simulink model "Lidar_System_July03_v2_noSave"  (Simulink 7.3)
settings: Solver=FixedStepDiscrete  StartTime=0.0  StopTime=inf  FixedStep=0.1  MaxStep=0.2  RelTol=1e-3
undefined symbols (not defined in the file): strel
libraries: dspmtrx3 x86, simulink x64, dspstat3 x37, vipstatistics x15, vipmorphops x15
(part 1 of 8)
settings Model: Creator=gclayton  LastModifiedBy=wildcat
settings DebuggingCC: InheritedTsInSrcMsg=none
settings RTWCC: SystemTargetFile=rlnx.tlc  GenCodeOnly=on  TemplateMakefile=rlnx_ubuntu.tmf  Description=Linux Real-Time Target  ProcessScript=rlnx_make_rtw_hook
settings RTWCC: CustomInclude=|
  | /usr/local/include/opencv/
  | /usr/local/include/
settings CodeAppCC: GenerateComments=off  SimulinkBlockComments=off
settings STFCustomTargetCC: ModelReferenceCompliant=off  MatFileLogging=on  SystemTargetFile=rlnx.tlc
settings GRTTargetCC: ModelReferenceCompliant=off  ParMdlRefBuildCompliant=off  CompOptLevelCompliant=off
settings CustomProperty: DataType=string  Value="-lm -ldl /usr/local/lib/libopencv_highgui.so.2.4 /usr/local/lib/libopencv_core.so.2.4 /usr/local/lib/libopencv_imgproc.so.2.4  -lc_urg -lc_urg_connection -lc_urg_system -lphidget21 -llcm"
settings EnumStrPairs: String=PC

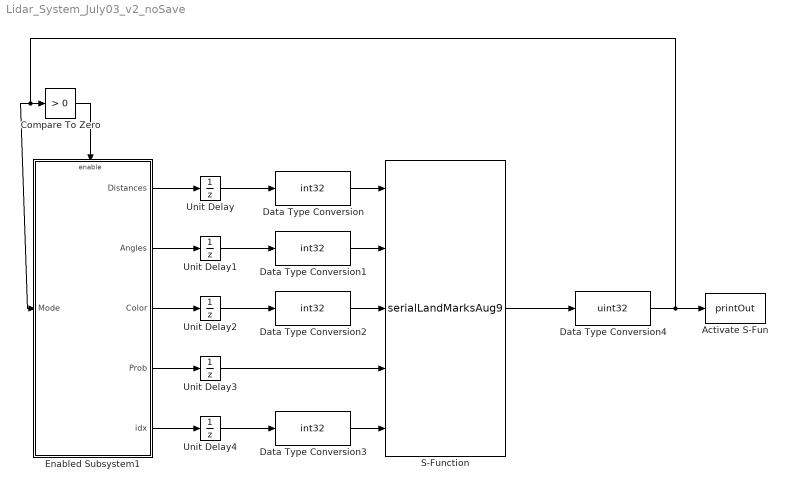
== system Lidar_System_July03_v2_noSave ==
  Activate S-Fun : S-Function  FunctionName=printOut  EnableBusSupport=off
  Compare To Zero : simulink/Logic and Bit Operations/Compare To Zero  SystemSampleTime=-1  relop=>  LogicOutDataTypeMode=uint8  ZeroCross=off
  Data Type Conversion{,1..3} (4 alike) : DataTypeConversion  OutDataTypeMode=int32  OutDataType=fixdt(1, 16)  OutScaling=2^0  OutDataTypeStr=int32
  Data Type Conversion4 : DataTypeConversion  OutDataTypeMode=uint32  OutDataType=fixdt(1, 16)  OutScaling=2^0  OutDataTypeStr=uint32
  Enabled Subsystem1 : Subsystem  TreatAsAtomicUnit=on
  S-Function : S-Function  FunctionName=serialLandMarksAug9  EnableBusSupport=off
  Unit Delay : UnitDelay  X0=zeros(1,12)  SampleTime=-1
  Unit Delay1 : UnitDelay  X0=zeros(1,12)  SampleTime=-1
  Unit Delay2 : UnitDelay  X0=zeros(4,1)  SampleTime=-1
  Unit Delay3 : UnitDelay  X0=zeros(4,1)  SampleTime=-1
  Unit Delay4 : UnitDelay  X0=zeros(4,1)  SampleTime=-1
  wires:
  Compare To Zero/1 -> Enabled Subsystem1/Enable
  Data Type Conversion4/1 -> Activate S-Fun/1, Compare To Zero/1, Enabled Subsystem1/1(Mode)
  S-Function/1 -> Data Type Conversion4/1
  Enabled Subsystem1/2(Angles) -> Unit Delay1/1
  Enabled Subsystem1/1(Distances) -> Unit Delay/1
  Enabled Subsystem1/3(Color) -> Unit Delay2/1
  Enabled Subsystem1/4(Prob) -> Unit Delay3/1
  Enabled Subsystem1/5(idx) -> Unit Delay4/1
  Unit Delay/1 -> Data Type Conversion/1
  Unit Delay1/1 -> Data Type Conversion1/1
  Unit Delay2/1 -> Data Type Conversion2/1
  Unit Delay4/1 -> Data Type Conversion3/1
  Data Type Conversion/1 -> S-Function/1
  Data Type Conversion1/1 -> S-Function/2
  Data Type Conversion2/1 -> S-Function/3
  Unit Delay3/1 -> S-Function/4
  Data Type Conversion3/1 -> S-Function/5

== system Lidar_System_July03_v2_noSave/Enabled Subsystem1 ==
  Mode : Inport  OutDataType=fixdt(1, 16)  OutScaling=2^0
  Enable : EnablePort
  Data Type Conversion : DataTypeConversion  OutDataTypeMode=int32  OutDataType=fixdt(1, 16)  OutScaling=2^0  OutDataTypeStr=int32
  Down Angle : Constant  Value=-25  OutDataType=fixdt(1, 16)  OutScaling=2^0
  Embedded MATLAB Function : Stateflow chart  TreatAsAtomicUnit=on
  Perception : Subsystem  TreatAsAtomicUnit=on
  S-Function : S-Function  FunctionName=TT_pot_readerV4  EnableBusSupport=off
  Scan Number (max 65) : Constant  Value=65  OutDataType=fixdt(1, 16)  OutScaling=2^0
  Sensing : S-Function  FunctionName=lidarCam_Select_June30_15  EnableBusSupport=off
  Sensor Enable : Stateflow chart  TreatAsAtomicUnit=on
  Stepper Speed and Postion  Calculation : Stateflow chart  TreatAsAtomicUnit=on
  Up Angle : Constant  Value=30  OutDataType=fixdt(1, 16)  OutScaling=2^0
  Distances : Outport  OutDataType=fixdt(1, 16)  OutScaling=2^0
  Angles : Outport  Port=2  OutDataType=fixdt(1, 16)  OutScaling=2^0
  Color : Outport  Port=3  OutDataType=fixdt(1, 16)  OutScaling=2^0
  Prob : Outport  Port=4  OutDataType=fixdt(1, 16)  OutScaling=2^0
  idx : Outport  Port=5  OutDataType=fixdt(1, 16)  OutScaling=2^0
  wires:
  Embedded MATLAB Function/1(yn) -> Perception/Enable
  Sensing/1 -> Perception/2(LidarData)
  Sensing/5 -> Perception/6(UpDown)
  Sensing/2 -> Perception/3(Red)
  Sensing/3 -> Perception/4(Green)
  Sensing/4 -> Perception/5(Blue)
  Mode/1 -> Perception/1(Mode), Sensor Enable/1(mode)
  Down Angle/1 -> Stepper Speed and Postion  Calculation/2(DownAngle)
  Up Angle/1 -> Stepper Speed and Postion  Calculation/1(UpAngle)
  Scan Number (max 65)/1 -> Stepper Speed and Postion  Calculation/3(Scans)
  Stepper Speed and Postion  Calculation/1(Speed) -> Sensing/3
  Stepper Speed and Postion  Calculation/2(Upos) -> Sensing/4
  Stepper Speed and Postion  Calculation/3(Dpos) -> Sensing/5
  Stepper Speed and Postion  Calculation/4(ScanNum) -> Sensing/6
  S-Function/1 -> Embedded MATLAB Function/1(potVal), Sensing/2
  Sensor Enable/1(choice) -> Data Type Conversion/1
  Data Type Conversion/1 -> Sensing/1
  Perception/1(Distances) -> Distances/1
  Perception/2(Angles) -> Angles/1
  Perception/3(Color) -> Color/1
  Perception/4(Prob) -> Prob/1
  Perception/5(idx) -> idx/1

== system Lidar_System_July03_v2_noSave/Enabled Subsystem1/Perception ==
  Mode : Inport  OutDataType=fixdt(1, 16)  OutScaling=2^0
  LidarData : Inport  Port=2  OutDataType=fixdt(1, 16)  OutScaling=2^0
  Red : Inport  Port=3  OutDataType=fixdt(1, 16)  OutScaling=2^0
  Green : Inport  Port=4  OutDataType=fixdt(1, 16)  OutScaling=2^0
  Blue : Inport  Port=5  OutDataType=fixdt(1, 16)  OutScaling=2^0
  UpDown : Inport  Port=6  OutDataType=fixdt(1, 16)  OutScaling=2^0
  Enable : EnablePort
  Bus Creator : BusCreator  Inputs=3
  Color Analysis : Subsystem
  Detect Landmarks : Subsystem
  Lidar data selector : Stateflow chart  TreatAsAtomicUnit=on
  Match Landmarks : Stateflow chart  TreatAsAtomicUnit=on
  Raster Image : Stateflow chart  TreatAsAtomicUnit=on
  Raster to UV scatter : Stateflow chart  TreatAsAtomicUnit=on
  Raster to UV scatter1 : Stateflow chart  TreatAsAtomicUnit=on
  S-Function4 : S-Function  FunctionName=rgbtohsv_sfunV2  EnableBusSupport=off
  Distances : Outport  OutDataType=fixdt(1, 16)  OutScaling=2^0
  Angles : Outport  Port=2  OutDataType=fixdt(1, 16)  OutScaling=2^0
  Color : Outport  Port=3  OutDataType=fixdt(1, 16)  OutScaling=2^0
  Prob : Outport  Port=4  OutDataType=fixdt(1, 16)  OutScaling=2^0
  idx : Outport  Port=5  OutDataType=fixdt(1, 16)  OutScaling=2^0
  wires:
  Lidar data selector/1(lidarOut) -> Raster Image/1(lidarData)
  Red/1 -> S-Function4/1
  Green/1 -> S-Function4/2
  Blue/1 -> S-Function4/3
  LidarData/1 -> Lidar data selector/1(lidarIn)
  S-Function4/1 -> Bus Creator/1  "H"
  S-Function4/2 -> Bus Creator/2  "S"
  S-Function4/3 -> Bus Creator/3  "V"
  Bus Creator/1 -> Color Analysis/3(HSV)
  Raster to UV scatter/1(depthImage) -> Color Analysis/2(uv_d)
  Mode/1 -> Color Analysis/1(Mode)
  Color Analysis/2(Prob) -> Prob/1
  Color Analysis/1(Color) -> Color/1
  Color Analysis/3(im_distances) -> Match Landmarks/1(im_distances)
  Color Analysis/4(im_angles) -> Match Landmarks/2(im_angles)
  Detect Landmarks/1(Distances) -> Match Landmarks/3(Distances)
  Detect Landmarks/2(Angles) -> Match Landmarks/4(Angles)
  Raster Image/1(dist_image) -> Raster to UV scatter1/1(DistIM), Detect Landmarks/1(dist_im)
  Raster to UV scatter1/1(scanAngle) -> Raster to UV scatter/1(scanAngle)
  Raster to UV scatter1/2(gimbalAngle) -> Raster to UV scatter/2(gimbalAngle)
  Raster to UV scatter1/3(range) -> Raster to UV scatter/3(range)
  Match Landmarks/1(idx) -> idx/1
  Match Landmarks/2(distances) -> Distances/1
  Match Landmarks/3(angles) -> Angles/1
  UpDown/1 -> Raster to UV scatter/4(upScan), Raster Image/2(UpDown)

== system Lidar_System_July03_v2_noSave/Enabled Subsystem1/Perception/Color Analysis ==
  Mode : Inport  OutDataType=fixdt(1, 16)  OutScaling=2^0
  uv_d : Inport  Port=2  OutDataType=fixdt(1, 16)  OutScaling=2^0
  HSV : Inport  Port=3  OutDataType=fixdt(1, 16)  OutScaling=2^0
  Acoustics (Empty) : Subsystem  TreatAsAtomicUnit=on
  Bus Selector : BusSelector  OutputSignals=Color,Prob,im_distances,im_angles
  Find Can Buoys : Subsystem  TreatAsAtomicUnit=on
  Light Buoy : Subsystem  TreatAsAtomicUnit=on
  Multiport Switch : MultiPortSwitch  Inputs=5  OutDataType=fixdt(1, 16)  OutScaling=2^0
  No Color Analysis1 : Subsystem  TreatAsAtomicUnit=on
  Switch Case : SwitchCase  CaseConditions={1,2,3,4}
  Template Matching (Docking) : Subsystem  TreatAsAtomicUnit=on
  Color : Outport  OutDataType=fixdt(1, 16)  OutScaling=2^0
  Prob : Outport  Port=2  OutDataType=fixdt(1, 16)  OutScaling=2^0
  im_distances : Outport  Port=3  OutDataType=fixdt(1, 16)  OutScaling=2^0
  im_angles : Outport  Port=4  OutDataType=fixdt(1, 16)  OutScaling=2^0
  wires:
  Mode/1 -> Switch Case/1, Multiport Switch/1, Template Matching (Docking)/3(mode)
  Find Can Buoys/1(Output) -> Multiport Switch/2
  Acoustics (Empty)/1(Output) -> Multiport Switch/3
  Bus Selector/1 -> Color/1  "<Color>"
  Bus Selector/2 -> Prob/1  "<Prob>"
  Bus Selector/3 -> im_distances/1  "<im_distances>"
  Bus Selector/4 -> im_angles/1  "<im_angles>"
  Template Matching (Docking)/1(Output) -> Multiport Switch/6
  Multiport Switch/1 -> Bus Selector/1
  Light Buoy/1(Output) -> Multiport Switch/4
  No Color Analysis1/1(Output) -> Multiport Switch/5
  Switch Case/1 -> Find Can Buoys/Action
  Switch Case/2 -> Acoustics (Empty)/Action
  Switch Case/3 -> Light Buoy/Action
  Switch Case/4 -> No Color Analysis1/Action
  uv_d/1 -> Find Can Buoys/1(uv_d), Acoustics (Empty)/1(uv_d), Light Buoy/1(uv_d), No Color Analysis1/1(uv_d), Template Matching (Docking)/1(uv_d)
  HSV/1 -> Light Buoy/2(HSV), No Color Analysis1/2(HSV), Template Matching (Docking)/2(HSV), Acoustics (Empty)/2(HSV), Find Can Buoys/2(HSV)
  Switch Case/5 -> Template Matching (Docking)/Action

== system Lidar_System_July03_v2_noSave/Enabled Subsystem1/Perception/Detect Landmarks ==
  dist_im : Inport  OutDataType=fixdt(1, 16)  OutScaling=2^0
  Blob Analysis : vipstatistics/Blob Analysis  Tag=vipblks_row_conv  DialogController=vipDDGCreate  DialogControllerArgs=DataTag51  area=off  centroid=on  bBox=on  majorAxis=off  minorAxis=off  angle=off  eccentricity=off  equivDiameterSq=off  extent=off  perimeter=off  maxBlobs=12  warnIfNumBlobsExceeded=on  isCount=off  useMinArea=on  minArea=30  useMaxArea=off  maxArea=intmax('uint32')  excludeBorderBlob=on  outDT=double  isOutVarDim=off  isFill=on  fillValues=-1  conn=8  isLabel=off  outputMode=Binary point scaling  outputWordLength=32  outputFracLength=16  firstCoeffMode=Binary point scaling  firstCoeffWordLength=16  firstCoeffFracLength=14  secondCoeffMode=Binary point scaling  secondCoeffWordLength=32  secondCoeffFracLength=16  accumMode=Binary point scaling  accumWordLength=32  accumFracLength=0  prodOutputMode=Binary point scaling  prodOutputWordLength=32  prodOutputFracLength=16  roundingMode=Floor  overflowMode=off
  Closing : vipmorphops/Closing  nhoodsrc=Specify via dialog  strel=strel('rectangle',[5 7])
  Embedded MATLAB Function1 : Stateflow chart  TreatAsAtomicUnit=on
  Logical Operator : Logic  AllPortsSameDT=off  OutDataTypeMode=boolean  LogicDataType=fixdt(0, 8)  OutDataTypeStr=boolean
  Max Thresh : simulink/Logic and Bit Operations/Compare To Constant  SystemSampleTime=-1  relop=<=  const=10000  LogicOutDataTypeMode=boolean  ZeroCross=off
  Min Thresh (removes pontoons) : simulink/Logic and Bit Operations/Compare To Constant  SystemSampleTime=-1  relop=>  const=2000  LogicOutDataTypeMode=boolean  ZeroCross=off
  Distances : Outport  OutDataType=fixdt(1, 16)  OutScaling=2^0
  Angles : Outport  Port=2  OutDataType=fixdt(1, 16)  OutScaling=2^0
  wires:
  Max Thresh/1 -> Logical Operator/1
  Min Thresh (removes pontoons)/1 -> Logical Operator/2
  dist_im/1 -> Max Thresh/1, Min Thresh (removes pontoons)/1, Embedded MATLAB Function1/4(dist_im)
  Embedded MATLAB Function1/1(Distances) -> Distances/1
  Embedded MATLAB Function1/2(Angles) -> Angles/1
  Logical Operator/1 -> Closing/1, Embedded MATLAB Function1/3(BW)
  Closing/1 -> Blob Analysis/1
  Blob Analysis/1 -> Embedded MATLAB Function1/1(centroid)
  Blob Analysis/2 -> Embedded MATLAB Function1/2(bbox)

== system Lidar_System_July03_v2_noSave/Enabled Subsystem1/Perception/Color Analysis/Acoustics (Empty) ==
  uv_d : Inport  OutDataType=fixdt(1, 16)  OutScaling=2^0
  HSV : Inport  Port=2  OutDataType=fixdt(1, 16)  OutScaling=2^0
  Action Port : ActionPort  ActionType=case
  Bus Creator : BusCreator
  Constant{,1..3} (4 alike) : Constant  Value=zeros(4,1)  OutDataType=fixdt(1, 16)  OutScaling=2^0
  Terminator : Terminator
  Terminator1 : Terminator
  Output : Outport  OutDataType=fixdt(1, 16)  OutScaling=2^0
  wires:
  uv_d/1 -> Terminator/1
  HSV/1 -> Terminator1/1
  Bus Creator/1 -> Output/1
  Constant3/1 -> Bus Creator/4  "im_angles"
  Constant2/1 -> Bus Creator/3  "im_distances"
  Constant1/1 -> Bus Creator/2  "Prob"
  Constant/1 -> Bus Creator/1  "Color"

== system Lidar_System_July03_v2_noSave/Enabled Subsystem1/Perception/Color Analysis/Find Can Buoys ==
  uv_d : Inport  OutDataType=fixdt(1, 16)  OutScaling=2^0
  HSV : Inport  Port=2  OutDataType=fixdt(1, 16)  OutScaling=2^0
  Action Port : ActionPort  ActionType=case
  Blob Analysis : vipstatistics/Blob Analysis  Tag=vipblks_row_conv  DialogController=vipDDGCreate  DialogControllerArgs=DataTag0  area=off  centroid=on  bBox=on  majorAxis=off  minorAxis=off  angle=off  eccentricity=off  equivDiameterSq=off  extent=off  perimeter=off  maxBlobs=12  warnIfNumBlobsExceeded=on  isCount=off  useMinArea=on  minArea=20  useMaxArea=off  maxArea=intmax('uint32')  excludeBorderBlob=on  outDT=double  isOutVarDim=off  isFill=on  fillValues=-1  conn=8  isLabel=off  outputMode=Binary point scaling  outputWordLength=32  outputFracLength=16  firstCoeffMode=Binary point scaling  firstCoeffWordLength=16  firstCoeffFracLength=14  secondCoeffMode=Binary point scaling  secondCoeffWordLength=32  secondCoeffFracLength=16  accumMode=Binary point scaling  accumWordLength=32  accumFracLength=0  prodOutputMode=Binary point scaling  prodOutputWordLength=32  prodOutputFracLength=16  roundingMode=Floor  overflowMode=off
  Bus Creator : BusCreator
  Bus Selector : BusSelector  OutputSignals=H
  Closing : vipmorphops/Closing  nhoodsrc=Specify via dialog  strel=strel('rectangle',[10 14])
  Constant1 : Constant  Value=zeros(4,1)  OutDataType=fixdt(1, 16)  OutScaling=2^0
  Embedded MATLAB Function1 : Stateflow chart  TreatAsAtomicUnit=on
  Logical Operator : Logic  AllPortsSameDT=off  OutDataTypeMode=boolean  LogicDataType=fixdt(0, 8)  OutDataTypeStr=boolean
  Max Thresh : simulink/Logic and Bit Operations/Compare To Constant  SystemSampleTime=-1  relop=<=  const=10000  LogicOutDataTypeMode=boolean  ZeroCross=off
  Min Thresh (removes pontoons) : simulink/Logic and Bit Operations/Compare To Constant  SystemSampleTime=-1  relop=>  const=2000  LogicOutDataTypeMode=boolean  ZeroCross=off
  Output : Outport  OutDataType=fixdt(1, 16)  OutScaling=2^0
  wires:
  Embedded MATLAB Function1/1(meanHues) -> Bus Creator/1  "Color"
  Constant1/1 -> Bus Creator/2  "Prob"
  Embedded MATLAB Function1/2(Distances) -> Bus Creator/3  "im_distances"
  Embedded MATLAB Function1/3(Angles) -> Bus Creator/4  "im_angles"
  Bus Creator/1 -> Output/1
  Max Thresh/1 -> Logical Operator/1
  Min Thresh (removes pontoons)/1 -> Logical Operator/2
  Logical Operator/1 -> Closing/1, Embedded MATLAB Function1/4(BW)
  Closing/1 -> Blob Analysis/1
  uv_d/1 -> Max Thresh/1, Min Thresh (removes pontoons)/1, Embedded MATLAB Function1/5(dist_im)
  Blob Analysis/1 -> Embedded MATLAB Function1/2(centroid)
  Blob Analysis/2 -> Embedded MATLAB Function1/3(bbox)
  HSV/1 -> Bus Selector/1
  Bus Selector/1 -> Embedded MATLAB Function1/1(H)  "<H>"

== system Lidar_System_July03_v2_noSave/Enabled Subsystem1/Perception/Color Analysis/Light Buoy ==
  uv_d : Inport  OutDataType=fixdt(1, 16)  OutScaling=2^0
  HSV : Inport  Port=2  OutDataType=fixdt(1, 16)  OutScaling=2^0
  Action Port : ActionPort  ActionType=case
  Bus Creator : BusCreator
  Bus Selector : BusSelector  OutputSignals=H,S,V
  Color Detection : Subsystem
  Constant1 : Constant  Value=zeros(4,1)  OutDataType=fixdt(1, 16)  OutScaling=2^0
  Constant2 : Constant  Value=zeros(4,1)  OutDataType=fixdt(1, 16)  OutScaling=2^0
  Constant3 : Constant  Value=zeros(4,1)  OutDataType=fixdt(1, 16)  OutScaling=2^0
  Format : Stateflow chart  TreatAsAtomicUnit=on
  Terminator : Terminator
  Output : Outport  OutDataType=fixdt(1, 16)  OutScaling=2^0
  wires:
  Color Detection/1(ColorOut) -> Format/1(ColorOut)
  Bus Selector/3 -> Color Detection/3(Vin)  "<V>"
  Bus Selector/2 -> Color Detection/2(Sin)  "<S>"
  Bus Selector/1 -> Color Detection/1(Hin)  "<H>"
  HSV/1 -> Bus Selector/1
  uv_d/1 -> Terminator/1
  Bus Creator/1 -> Output/1
  Constant3/1 -> Bus Creator/4  "im_angles"
  Constant2/1 -> Bus Creator/3  "im_distances"
  Constant1/1 -> Bus Creator/2  "Prob"
  Format/1(Color) -> Bus Creator/1  "Color"

== system Lidar_System_July03_v2_noSave/Enabled Subsystem1/Perception/Color Analysis/No Color Analysis1 ==
  uv_d : Inport  OutDataType=fixdt(1, 16)  OutScaling=2^0
  HSV : Inport  Port=2  OutDataType=fixdt(1, 16)  OutScaling=2^0
  Action Port : ActionPort  ActionType=case
  Bus Creator : BusCreator
  Constant{,1..3} (4 alike) : Constant  Value=zeros(4,1)  OutDataType=fixdt(1, 16)  OutScaling=2^0
  Terminator : Terminator
  Terminator1 : Terminator
  Output : Outport  OutDataType=fixdt(1, 16)  OutScaling=2^0
  wires:
  Constant/1 -> Bus Creator/1  "Color"
  Constant1/1 -> Bus Creator/2  "Prob"
  Constant2/1 -> Bus Creator/3  "im_distances"
  Constant3/1 -> Bus Creator/4  "im_angles"
  Bus Creator/1 -> Output/1
  HSV/1 -> Terminator1/1
  uv_d/1 -> Terminator/1

== system Lidar_System_July03_v2_noSave/Enabled Subsystem1/Perception/Color Analysis/Template Matching (Docking) ==
  uv_d : Inport  OutDataType=fixdt(1, 16)  OutScaling=2^0
  HSV : Inport  Port=2  OutDataType=fixdt(1, 16)  OutScaling=2^0
  mode : Inport  Port=3  OutDataType=fixdt(1, 16)  OutScaling=2^0
  Action Port : ActionPort  ActionType=default
  Black : Subsystem
  Blue : Subsystem
  Embedded MATLAB Function : Stateflow chart
  Green : Subsystem
  Multiport Switch : MultiPortSwitch  Inputs=4  OutDataType=fixdt(1, 16)  OutScaling=2^0
  Red : Subsystem
  Output : Outport  OutDataType=fixdt(1, 16)  OutScaling=2^0
  wires:
  uv_d/1 -> Red/3(uv_d), Green/3(uv_d), Blue/3(uv_d), Black/3(uv_d)
  HSV/1 -> Green/2(HSV), Blue/2(HSV), Black/2(HSV), Red/2(HSV)
  mode/1 -> Embedded MATLAB Function/1(mode), Multiport Switch/1, Red/1(mode), Green/1(mode), Blue/1(mode), Black/1(mode)
  Red/1(Output1) -> Multiport Switch/2
  Multiport Switch/1 -> Output/1
  Embedded MATLAB Function/1(RedEn) -> Red/Enable
  Blue/1(Output1) -> Multiport Switch/4
  Green/1(Output1) -> Multiport Switch/3
  Embedded MATLAB Function/2(GreenEn) -> Green/Enable
  Embedded MATLAB Function/3(BlueEn) -> Blue/Enable
  Embedded MATLAB Function/4(BlackEn) -> Black/Enable
  Black/1(Output1) -> Multiport Switch/5

== system Lidar_System_July03_v2_noSave/Enabled Subsystem1/Perception/Color Analysis/Light Buoy/Color Detection ==
  Hin : Inport  OutDataType=fixdt(1, 16)  OutScaling=2^0
  Sin : Inport  Port=2  OutDataType=fixdt(1, 16)  OutScaling=2^0
  Vin : Inport  Port=3  OutDataType=fixdt(1, 16)  OutScaling=2^0
  Closing : vipmorphops/Closing  nhoodsrc=Specify via dialog  strel=strel('square',12)
  Embedded MATLAB Function : Stateflow chart  TreatAsAtomicUnit=on
  Find Bounding Box : Subsystem
  H Limit : simulink/Logic and Bit Operations/Compare To Constant  SystemSampleTime=-1  relop=>  const=60  LogicOutDataTypeMode=uint8  ZeroCross=off
  Logical Operator : Logic  AllPortsSameDT=off  OutDataTypeMode=boolean  LogicDataType=fixdt(0, 8)  OutDataTypeStr=boolean
  S Limit : simulink/Logic and Bit Operations/Compare To Constant  SystemSampleTime=-1  relop=>  const=144  LogicOutDataTypeMode=uint8  ZeroCross=off
  S-Function : S-Function  FunctionName=BuoyColorSeq  EnableBusSupport=off
  ColorOut : Outport  OutDataType=fixdt(1, 16)  OutScaling=2^0
  wires:
  S-Function/1 -> ColorOut/1
  Embedded MATLAB Function/1(ColorOut) -> S-Function/1
  Hin/1 -> Embedded MATLAB Function/2(Hin)
  Find Bounding Box/1(BBox) -> Embedded MATLAB Function/1(BBox)
  Closing/1 -> Find Bounding Box/1(BW_im)
  Logical Operator/1 -> Closing/1
  H Limit/1 -> Logical Operator/2
  S Limit/1 -> Logical Operator/1
  Vin/1 -> H Limit/1
  Sin/1 -> S Limit/1

== system Lidar_System_July03_v2_noSave/Enabled Subsystem1/Perception/Color Analysis/Template Matching (Docking)/Black ==
  mode : Inport  OutDataType=fixdt(1, 16)  OutScaling=2^0
  HSV : Inport  Port=2  OutDataType=fixdt(1, 16)  OutScaling=2^0
  uv_d : Inport  Port=3  OutDataType=fixdt(1, 16)  OutScaling=2^0
  Enable : EnablePort
  Circle : Subsystem
  Cruciform : Subsystem
  Embedded MATLAB Function : Stateflow chart
  Multiport Switch : MultiPortSwitch  OutDataType=fixdt(1, 16)  OutScaling=2^0
  Triangle : Subsystem
  Output1 : Outport  OutDataType=fixdt(1, 16)  OutScaling=2^0
  wires:
  mode/1 -> Multiport Switch/1, Embedded MATLAB Function/1(mode)
  Multiport Switch/1 -> Output1/1
  uv_d/1 -> Cruciform/1(uv_d), Circle/1(uv_d), Triangle/1(uv_d)
  HSV/1 -> Triangle/2(HSV), Circle/2(HSV), Cruciform/2(HSV)
  Cruciform/1(Output) -> Multiport Switch/2
  Circle/1(Output) -> Multiport Switch/3
  Triangle/1(Output) -> Multiport Switch/4
  Embedded MATLAB Function/1(CrucEn) -> Cruciform/Enable
  Embedded MATLAB Function/2(CircleEn) -> Circle/Enable
  Embedded MATLAB Function/3(TriEn) -> Triangle/Enable

== system Lidar_System_July03_v2_noSave/Enabled Subsystem1/Perception/Color Analysis/Template Matching (Docking)/Blue ==
  mode : Inport  OutDataType=fixdt(1, 16)  OutScaling=2^0
  HSV : Inport  Port=2  OutDataType=fixdt(1, 16)  OutScaling=2^0
  uv_d : Inport  Port=3  OutDataType=fixdt(1, 16)  OutScaling=2^0
  Enable : EnablePort
  Circle : Subsystem
  Cruciform : Subsystem
  Embedded MATLAB Function : Stateflow chart
  Multiport Switch : MultiPortSwitch  OutDataType=fixdt(1, 16)  OutScaling=2^0
  Triangle : Subsystem
  Output1 : Outport  OutDataType=fixdt(1, 16)  OutScaling=2^0
  wires:
  mode/1 -> Multiport Switch/1, Embedded MATLAB Function/1(mode)
  Multiport Switch/1 -> Output1/1
  uv_d/1 -> Cruciform/1(uv_d), Circle/1(uv_d), Triangle/1(uv_d)
  HSV/1 -> Triangle/2(HSV), Circle/2(HSV), Cruciform/2(HSV)
  Cruciform/1(Output) -> Multiport Switch/2
  Circle/1(Output) -> Multiport Switch/3
  Triangle/1(Output) -> Multiport Switch/4
  Embedded MATLAB Function/1(CrucEn) -> Cruciform/Enable
  Embedded MATLAB Function/2(CircleEn) -> Circle/Enable
  Embedded MATLAB Function/3(TriEn) -> Triangle/Enable

== system Lidar_System_July03_v2_noSave/Enabled Subsystem1/Perception/Color Analysis/Template Matching (Docking)/Green ==
  mode : Inport  OutDataType=fixdt(1, 16)  OutScaling=2^0
  HSV : Inport  Port=2  OutDataType=fixdt(1, 16)  OutScaling=2^0
  uv_d : Inport  Port=3  OutDataType=fixdt(1, 16)  OutScaling=2^0
  Enable : EnablePort
  Circle : Subsystem
  Cruciform : Subsystem
  Embedded MATLAB Function : Stateflow chart
  Multiport Switch : MultiPortSwitch  OutDataType=fixdt(1, 16)  OutScaling=2^0
  Triangle : Subsystem
  Output1 : Outport  OutDataType=fixdt(1, 16)  OutScaling=2^0
  wires:
  mode/1 -> Multiport Switch/1, Embedded MATLAB Function/1(mode)
  Multiport Switch/1 -> Output1/1
  Triangle/1(Output) -> Multiport Switch/4
  Circle/1(Output) -> Multiport Switch/3
  Cruciform/1(Output) -> Multiport Switch/2
  uv_d/1 -> Cruciform/1(uv_d), Circle/1(uv_d), Triangle/1(uv_d)
  HSV/1 -> Triangle/2(HSV), Circle/2(HSV), Cruciform/2(HSV)
  Embedded MATLAB Function/2(CircleEn) -> Circle/Enable
  Embedded MATLAB Function/1(CrucEn) -> Cruciform/Enable
  Embedded MATLAB Function/3(TriEn) -> Triangle/Enable

== system Lidar_System_July03_v2_noSave/Enabled Subsystem1/Perception/Color Analysis/Template Matching (Docking)/Red ==
  mode : Inport  OutDataType=fixdt(1, 16)  OutScaling=2^0
  HSV : Inport  Port=2  OutDataType=fixdt(1, 16)  OutScaling=2^0
  uv_d : Inport  Port=3  OutDataType=fixdt(1, 16)  OutScaling=2^0
  Enable : EnablePort
  Circle : Subsystem
  Cruciform : Subsystem
  Embedded MATLAB Function : Stateflow chart
  Multiport Switch : MultiPortSwitch  OutDataType=fixdt(1, 16)  OutScaling=2^0
  Triangle : Subsystem
  Output1 : Outport  OutDataType=fixdt(1, 16)  OutScaling=2^0
  wires:
  mode/1 -> Multiport Switch/1, Embedded MATLAB Function/1(mode)
  Multiport Switch/1 -> Output1/1
  Cruciform/1(Output) -> Multiport Switch/2
  Circle/1(Output) -> Multiport Switch/3
  Triangle/1(Output) -> Multiport Switch/4
  uv_d/1 -> Cruciform/1(uv_d), Circle/1(uv_d), Triangle/1(uv_d)
  HSV/1 -> Cruciform/2(HSV), Circle/2(HSV), Triangle/2(HSV)
  Embedded MATLAB Function/1(CrucEn) -> Cruciform/Enable
  Embedded MATLAB Function/2(CircleEn) -> Circle/Enable
  Embedded MATLAB Function/3(TriEn) -> Triangle/Enable

== system Lidar_System_July03_v2_noSave/Enabled Subsystem1/Perception/Color Analysis/Light Buoy/Color Detection/Find Bounding Box ==
  BW_im : Inport
  Blob Analysis : vipstatistics/Blob Analysis  Tag=vipblks_row_conv  DialogController=vipDDGCreate  DialogControllerArgs=DataTag1  area=on  centroid=off  bBox=on  majorAxis=off  minorAxis=off  angle=off  eccentricity=off  equivDiameterSq=off  extent=off  perimeter=off  maxBlobs=4  warnIfNumBlobsExceeded=on  isCount=off  useMinArea=on  minArea=30  useMaxArea=off  maxArea=intmax('uint32')  excludeBorderBlob=off  outDT=double  isOutVarDim=off  isFill=on  fillValues=-1  conn=8  isLabel=off  outputMode=Binary point scaling  outputWordLength=32  outputFracLength=16  firstCoeffMode=Binary point scaling  firstCoeffWordLength=16  firstCoeffFracLength=14  secondCoeffMode=Binary point scaling  secondCoeffWordLength=32  secondCoeffFracLength=16  accumMode=Binary point scaling  accumWordLength=32  accumFracLength=0  prodOutputMode=Binary point scaling  prodOutputWordLength=32  prodOutputFracLength=16  roundingMode=Floor  overflowMode=off
  Permute Matrix : dspmtrx3/Permute Matrix  mode=Columns  ZeroOneIdxMode=One-based  errmode=Clip index  checkDims=off
  Sort : dspstat3/Sort  DialogController=dspDDGCreate  DialogControllerArgs=DataTag2  otype=Index  dir=Descending  sortAlg=Quick sort  roundingMode=Floor  overflowMode=off
  Submatrix : dspmtrx3/Submatrix  RowSpan=All rows  RowStartMode=First  RowStartIndex=1  RowEndMode=Last  RowEndIndex=1  ColSpan=One column  ColStartMode=First  ColStartIndex=1  ColEndMode=Last  ColEndIndex=1
  BBox : Outport
  wires:
  Submatrix/1 -> BBox/1
  BW_im/1 -> Blob Analysis/1
  Permute Matrix/1 -> Submatrix/1
  Blob Analysis/2 -> Permute Matrix/1
  Sort/1 -> Permute Matrix/2
  Blob Analysis/1 -> Sort/1

== system Lidar_System_July03_v2_noSave/Enabled Subsystem1/Perception/Color Analysis/Template Matching (Docking)/Black/Circle ==
  uv_d : Inport  OutDataType=fixdt(1, 16)  OutScaling=2^0
  HSV : Inport  Port=2  OutDataType=fixdt(1, 16)  OutScaling=2^0
  Enable : EnablePort
  Bus Creator : BusCreator
  Bus Selector : BusSelector  OutputSignals=H,S,V
  Circle : Constant  Value=2  OutDataType=fixdt(1, 16)  OutScaling=2^0
  Constant : Constant  Value=zeros(4,1)  OutDataType=fixdt(1, 16)  OutScaling=2^0
  Constant1 : Constant  Value=zeros(4,1)  OutDataType=fixdt(1, 16)  OutScaling=2^0
  Docking1 : Subsystem
  Output : Outport  OutDataType=fixdt(1, 16)  OutScaling=2^0
  wires:
  uv_d/1 -> Docking1/5(uv_d)
  HSV/1 -> Bus Selector/1
  Bus Selector/3 -> Docking1/4(V)  "<V>"
  Bus Selector/2 -> Docking1/3(S)  "<S>"
  Bus Selector/1 -> Docking1/2(H)  "<H>"
  Circle/1 -> Docking1/1(Target)
  Bus Creator/1 -> Output/1
  Docking1/2(Angles) -> Bus Creator/4  "im_angles"
  Docking1/1(Distances) -> Bus Creator/3  "im_distances"
  Constant1/1 -> Bus Creator/2  "Prob"
  Constant/1 -> Bus Creator/1  "Color"

== system Lidar_System_July03_v2_noSave/Enabled Subsystem1/Perception/Color Analysis/Template Matching (Docking)/Black/Cruciform ==
  uv_d : Inport  OutDataType=fixdt(1, 16)  OutScaling=2^0
  HSV : Inport  Port=2  OutDataType=fixdt(1, 16)  OutScaling=2^0
  Enable : EnablePort
  Bus Creator : BusCreator
  Bus Selector : BusSelector  OutputSignals=H,S,V
  Constant : Constant  Value=zeros(4,1)  OutDataType=fixdt(1, 16)  OutScaling=2^0
  Constant1 : Constant  Value=zeros(4,1)  OutDataType=fixdt(1, 16)  OutScaling=2^0
  Cruciform : Constant  OutDataType=fixdt(1, 16)  OutScaling=2^0
  Docking1 : Subsystem
  Output : Outport  OutDataType=fixdt(1, 16)  OutScaling=2^0
  wires:
  uv_d/1 -> Docking1/5(uv_d)
  HSV/1 -> Bus Selector/1
  Bus Selector/3 -> Docking1/4(V)  "<V>"
  Bus Selector/2 -> Docking1/3(S)  "<S>"
  Bus Selector/1 -> Docking1/2(H)  "<H>"
  Cruciform/1 -> Docking1/1(Target)
  Bus Creator/1 -> Output/1
  Docking1/2(Angles) -> Bus Creator/4  "im_angles"
  Docking1/1(Distances) -> Bus Creator/3  "im_distances"
  Constant1/1 -> Bus Creator/2  "Prob"
  Constant/1 -> Bus Creator/1  "Color"

== system Lidar_System_July03_v2_noSave/Enabled Subsystem1/Perception/Color Analysis/Template Matching (Docking)/Black/Triangle ==
  uv_d : Inport  OutDataType=fixdt(1, 16)  OutScaling=2^0
  HSV : Inport  Port=2  OutDataType=fixdt(1, 16)  OutScaling=2^0
  Enable : EnablePort
  Bus Creator : BusCreator
  Bus Selector : BusSelector  OutputSignals=H,S,V
  Constant : Constant  Value=zeros(4,1)  OutDataType=fixdt(1, 16)  OutScaling=2^0
  Constant1 : Constant  Value=zeros(4,1)  OutDataType=fixdt(1, 16)  OutScaling=2^0
  Docking1 : Subsystem
  Triangle : Constant  Value=3  OutDataType=fixdt(1, 16)  OutScaling=2^0
  Output : Outport  OutDataType=fixdt(1, 16)  OutScaling=2^0
  wires:
  uv_d/1 -> Docking1/5(uv_d)
  HSV/1 -> Bus Selector/1
  Bus Selector/3 -> Docking1/4(V)  "<V>"
  Bus Selector/2 -> Docking1/3(S)  "<S>"
  Bus Selector/1 -> Docking1/2(H)  "<H>"
  Triangle/1 -> Docking1/1(Target)
  Bus Creator/1 -> Output/1
  Docking1/2(Angles) -> Bus Creator/4  "im_angles"
  Docking1/1(Distances) -> Bus Creator/3  "im_distances"
  Constant1/1 -> Bus Creator/2  "Prob"
  Constant/1 -> Bus Creator/1  "Color"

== system Lidar_System_July03_v2_noSave/Enabled Subsystem1/Perception/Color Analysis/Template Matching (Docking)/Blue/Circle ==
  uv_d : Inport  OutDataType=fixdt(1, 16)  OutScaling=2^0
  HSV : Inport  Port=2  OutDataType=fixdt(1, 16)  OutScaling=2^0
  Enable : EnablePort
  Bus Creator : BusCreator
  Bus Selector : BusSelector  OutputSignals=H,S,V
  Circle : Constant  Value=2  OutDataType=fixdt(1, 16)  OutScaling=2^0
  Constant : Constant  Value=zeros(4,1)  OutDataType=fixdt(1, 16)  OutScaling=2^0
  Constant1 : Constant  Value=zeros(4,1)  OutDataType=fixdt(1, 16)  OutScaling=2^0
  Docking1 : Subsystem
  Output : Outport  OutDataType=fixdt(1, 16)  OutScaling=2^0
  wires:
  uv_d/1 -> Docking1/5(uv_d)
  HSV/1 -> Bus Selector/1
  Bus Selector/3 -> Docking1/4(V)  "<V>"
  Bus Selector/2 -> Docking1/3(S)  "<S>"
  Bus Selector/1 -> Docking1/2(H)  "<H>"
  Circle/1 -> Docking1/1(Target)
  Bus Creator/1 -> Output/1
  Docking1/2(Angles) -> Bus Creator/4  "im_angles"
  Docking1/1(Distances) -> Bus Creator/3  "im_distances"
  Constant1/1 -> Bus Creator/2  "Prob"
  Constant/1 -> Bus Creator/1  "Color"

== system Lidar_System_July03_v2_noSave/Enabled Subsystem1/Perception/Color Analysis/Template Matching (Docking)/Blue/Cruciform ==
  uv_d : Inport  OutDataType=fixdt(1, 16)  OutScaling=2^0
  HSV : Inport  Port=2  OutDataType=fixdt(1, 16)  OutScaling=2^0
  Enable : EnablePort
  Bus Creator : BusCreator
  Bus Selector : BusSelector  OutputSignals=H,S,V
  Constant : Constant  Value=zeros(4,1)  OutDataType=fixdt(1, 16)  OutScaling=2^0
  Constant1 : Constant  Value=zeros(4,1)  OutDataType=fixdt(1, 16)  OutScaling=2^0
  Cruciform : Constant  OutDataType=fixdt(1, 16)  OutScaling=2^0
  Docking1 : Subsystem
  Output : Outport  OutDataType=fixdt(1, 16)  OutScaling=2^0
  wires:
  uv_d/1 -> Docking1/5(uv_d)
  HSV/1 -> Bus Selector/1
  Bus Selector/3 -> Docking1/4(V)  "<V>"
  Bus Selector/2 -> Docking1/3(S)  "<S>"
  Bus Selector/1 -> Docking1/2(H)  "<H>"
  Cruciform/1 -> Docking1/1(Target)
  Bus Creator/1 -> Output/1
  Docking1/2(Angles) -> Bus Creator/4  "im_angles"
  Docking1/1(Distances) -> Bus Creator/3  "im_distances"
  Constant1/1 -> Bus Creator/2  "Prob"
  Constant/1 -> Bus Creator/1  "Color"

== system Lidar_System_July03_v2_noSave/Enabled Subsystem1/Perception/Color Analysis/Template Matching (Docking)/Blue/Triangle ==
  uv_d : Inport  OutDataType=fixdt(1, 16)  OutScaling=2^0
  HSV : Inport  Port=2  OutDataType=fixdt(1, 16)  OutScaling=2^0
  Enable : EnablePort
  Bus Creator : BusCreator
  Bus Selector : BusSelector  OutputSignals=H,S,V
  Constant : Constant  Value=zeros(4,1)  OutDataType=fixdt(1, 16)  OutScaling=2^0
  Constant1 : Constant  Value=zeros(4,1)  OutDataType=fixdt(1, 16)  OutScaling=2^0
  Docking1 : Subsystem
  Triangle : Constant  Value=3  OutDataType=fixdt(1, 16)  OutScaling=2^0
  Output : Outport  OutDataType=fixdt(1, 16)  OutScaling=2^0
  wires:
  uv_d/1 -> Docking1/5(uv_d)
  HSV/1 -> Bus Selector/1
  Bus Selector/3 -> Docking1/4(V)  "<V>"
  Bus Selector/2 -> Docking1/3(S)  "<S>"
  Bus Selector/1 -> Docking1/2(H)  "<H>"
  Triangle/1 -> Docking1/1(Target)
  Bus Creator/1 -> Output/1
  Docking1/2(Angles) -> Bus Creator/4  "im_angles"
  Docking1/1(Distances) -> Bus Creator/3  "im_distances"
  Constant1/1 -> Bus Creator/2  "Prob"
  Constant/1 -> Bus Creator/1  "Color"

== system Lidar_System_July03_v2_noSave/Enabled Subsystem1/Perception/Color Analysis/Template Matching (Docking)/Green/Circle ==
  uv_d : Inport  OutDataType=fixdt(1, 16)  OutScaling=2^0
  HSV : Inport  Port=2  OutDataType=fixdt(1, 16)  OutScaling=2^0
  Enable : EnablePort
  Bus Creator : BusCreator
  Bus Selector : BusSelector  OutputSignals=H,S,V
  Circle : Constant  Value=2  OutDataType=fixdt(1, 16)  OutScaling=2^0
  Constant : Constant  Value=zeros(4,1)  OutDataType=fixdt(1, 16)  OutScaling=2^0
  Constant1 : Constant  Value=zeros(4,1)  OutDataType=fixdt(1, 16)  OutScaling=2^0
  Docking1 : Subsystem
  Output : Outport  OutDataType=fixdt(1, 16)  OutScaling=2^0
  wires:
  uv_d/1 -> Docking1/5(uv_d)
  HSV/1 -> Bus Selector/1
  Bus Selector/3 -> Docking1/4(V)  "<V>"
  Bus Selector/2 -> Docking1/3(S)  "<S>"
  Bus Selector/1 -> Docking1/2(H)  "<H>"
  Circle/1 -> Docking1/1(Target)
  Bus Creator/1 -> Output/1
  Docking1/2(Angles) -> Bus Creator/4  "im_angles"
  Docking1/1(Distances) -> Bus Creator/3  "im_distances"
  Constant1/1 -> Bus Creator/2  "Prob"
  Constant/1 -> Bus Creator/1  "Color"

== system Lidar_System_July03_v2_noSave/Enabled Subsystem1/Perception/Color Analysis/Template Matching (Docking)/Green/Cruciform ==
  uv_d : Inport  OutDataType=fixdt(1, 16)  OutScaling=2^0
  HSV : Inport  Port=2  OutDataType=fixdt(1, 16)  OutScaling=2^0
  Enable : EnablePort
  Bus Creator : BusCreator
  Bus Selector : BusSelector  OutputSignals=H,S,V
  Constant : Constant  Value=zeros(4,1)  OutDataType=fixdt(1, 16)  OutScaling=2^0
  Constant1 : Constant  Value=zeros(4,1)  OutDataType=fixdt(1, 16)  OutScaling=2^0
  Cruciform : Constant  OutDataType=fixdt(1, 16)  OutScaling=2^0
  Docking1 : Subsystem
  Output : Outport  OutDataType=fixdt(1, 16)  OutScaling=2^0
  wires:
  uv_d/1 -> Docking1/5(uv_d)
  HSV/1 -> Bus Selector/1
  Bus Selector/3 -> Docking1/4(V)  "<V>"
  Bus Selector/2 -> Docking1/3(S)  "<S>"
  Bus Selector/1 -> Docking1/2(H)  "<H>"
  Cruciform/1 -> Docking1/1(Target)
  Bus Creator/1 -> Output/1
  Docking1/2(Angles) -> Bus Creator/4  "im_angles"
  Docking1/1(Distances) -> Bus Creator/3  "im_distances"
  Constant1/1 -> Bus Creator/2  "Prob"
  Constant/1 -> Bus Creator/1  "Color"

== system Lidar_System_July03_v2_noSave/Enabled Subsystem1/Perception/Color Analysis/Template Matching (Docking)/Green/Triangle ==
  uv_d : Inport  OutDataType=fixdt(1, 16)  OutScaling=2^0
  HSV : Inport  Port=2  OutDataType=fixdt(1, 16)  OutScaling=2^0
  Enable : EnablePort
  Bus Creator : BusCreator
  Bus Selector : BusSelector  OutputSignals=H,S,V
  Constant : Constant  Value=zeros(4,1)  OutDataType=fixdt(1, 16)  OutScaling=2^0
  Constant1 : Constant  Value=zeros(4,1)  OutDataType=fixdt(1, 16)  OutScaling=2^0
  Docking1 : Subsystem
  Triangle : Constant  Value=3  OutDataType=fixdt(1, 16)  OutScaling=2^0
  Output : Outport  OutDataType=fixdt(1, 16)  OutScaling=2^0
  wires:
  uv_d/1 -> Docking1/5(uv_d)
  HSV/1 -> Bus Selector/1
  Bus Selector/3 -> Docking1/4(V)  "<V>"
  Bus Selector/2 -> Docking1/3(S)  "<S>"
  Bus Selector/1 -> Docking1/2(H)  "<H>"
  Triangle/1 -> Docking1/1(Target)
  Bus Creator/1 -> Output/1
  Docking1/2(Angles) -> Bus Creator/4  "im_angles"
  Docking1/1(Distances) -> Bus Creator/3  "im_distances"
  Constant1/1 -> Bus Creator/2  "Prob"
  Constant/1 -> Bus Creator/1  "Color"

== system Lidar_System_July03_v2_noSave/Enabled Subsystem1/Perception/Color Analysis/Template Matching (Docking)/Red/Circle ==
  uv_d : Inport  OutDataType=fixdt(1, 16)  OutScaling=2^0
  HSV : Inport  Port=2  OutDataType=fixdt(1, 16)  OutScaling=2^0
  Enable : EnablePort
  Bus Creator : BusCreator
  Bus Selector : BusSelector  OutputSignals=H,S,V
  Circle : Constant  Value=2  OutDataType=fixdt(1, 16)  OutScaling=2^0
  Constant : Constant  Value=zeros(4,1)  OutDataType=fixdt(1, 16)  OutScaling=2^0
  Constant1 : Constant  Value=zeros(4,1)  OutDataType=fixdt(1, 16)  OutScaling=2^0
  Docking1 : Subsystem
  Output : Outport  OutDataType=fixdt(1, 16)  OutScaling=2^0
  wires:
  uv_d/1 -> Docking1/5(uv_d)
  HSV/1 -> Bus Selector/1
  Bus Selector/3 -> Docking1/4(V)  "<V>"
  Bus Selector/2 -> Docking1/3(S)  "<S>"
  Bus Selector/1 -> Docking1/2(H)  "<H>"
  Circle/1 -> Docking1/1(Target)
  Bus Creator/1 -> Output/1
  Docking1/2(Angles) -> Bus Creator/4  "im_angles"
  Docking1/1(Distances) -> Bus Creator/3  "im_distances"
  Constant1/1 -> Bus Creator/2  "Prob"
  Constant/1 -> Bus Creator/1  "Color"

== system Lidar_System_July03_v2_noSave/Enabled Subsystem1/Perception/Color Analysis/Template Matching (Docking)/Red/Cruciform ==
  uv_d : Inport  OutDataType=fixdt(1, 16)  OutScaling=2^0
  HSV : Inport  Port=2  OutDataType=fixdt(1, 16)  OutScaling=2^0
  Enable : EnablePort
  Bus Creator : BusCreator
  Bus Selector : BusSelector  OutputSignals=H,S,V
  Constant : Constant  Value=zeros(4,1)  OutDataType=fixdt(1, 16)  OutScaling=2^0
  Constant1 : Constant  Value=zeros(4,1)  OutDataType=fixdt(1, 16)  OutScaling=2^0
  Cruciform : Constant  OutDataType=fixdt(1, 16)  OutScaling=2^0
  Docking1 : Subsystem
  Output : Outport  OutDataType=fixdt(1, 16)  OutScaling=2^0
  wires:
  uv_d/1 -> Docking1/5(uv_d)
  HSV/1 -> Bus Selector/1
  Bus Selector/3 -> Docking1/4(V)  "<V>"
  Bus Selector/2 -> Docking1/3(S)  "<S>"
  Bus Selector/1 -> Docking1/2(H)  "<H>"
  Cruciform/1 -> Docking1/1(Target)
  Bus Creator/1 -> Output/1
  Docking1/2(Angles) -> Bus Creator/4  "im_angles"
  Docking1/1(Distances) -> Bus Creator/3  "im_distances"
  Constant1/1 -> Bus Creator/2  "Prob"
  Constant/1 -> Bus Creator/1  "Color"

== system Lidar_System_July03_v2_noSave/Enabled Subsystem1/Perception/Color Analysis/Template Matching (Docking)/Red/Triangle ==
  uv_d : Inport  OutDataType=fixdt(1, 16)  OutScaling=2^0
  HSV : Inport  Port=2  OutDataType=fixdt(1, 16)  OutScaling=2^0
  Enable : EnablePort
  Bus Creator : BusCreator
  Bus Selector : BusSelector  OutputSignals=H,S,V
  Constant : Constant  Value=zeros(4,1)  OutDataType=fixdt(1, 16)  OutScaling=2^0
  Constant1 : Constant  Value=zeros(4,1)  OutDataType=fixdt(1, 16)  OutScaling=2^0
  Docking1 : Subsystem
  Triangle : Constant  Value=3  OutDataType=fixdt(1, 16)  OutScaling=2^0
  Output : Outport  OutDataType=fixdt(1, 16)  OutScaling=2^0
  wires:
  uv_d/1 -> Docking1/5(uv_d)
  HSV/1 -> Bus Selector/1
  Bus Selector/3 -> Docking1/4(V)  "<V>"
  Bus Selector/2 -> Docking1/3(S)  "<S>"
  Bus Selector/1 -> Docking1/2(H)  "<H>"
  Triangle/1 -> Docking1/1(Target)
  Bus Creator/1 -> Output/1
  Docking1/2(Angles) -> Bus Creator/4  "im_angles"
  Docking1/1(Distances) -> Bus Creator/3  "im_distances"
  Constant1/1 -> Bus Creator/2  "Prob"
  Constant/1 -> Bus Creator/1  "Color"

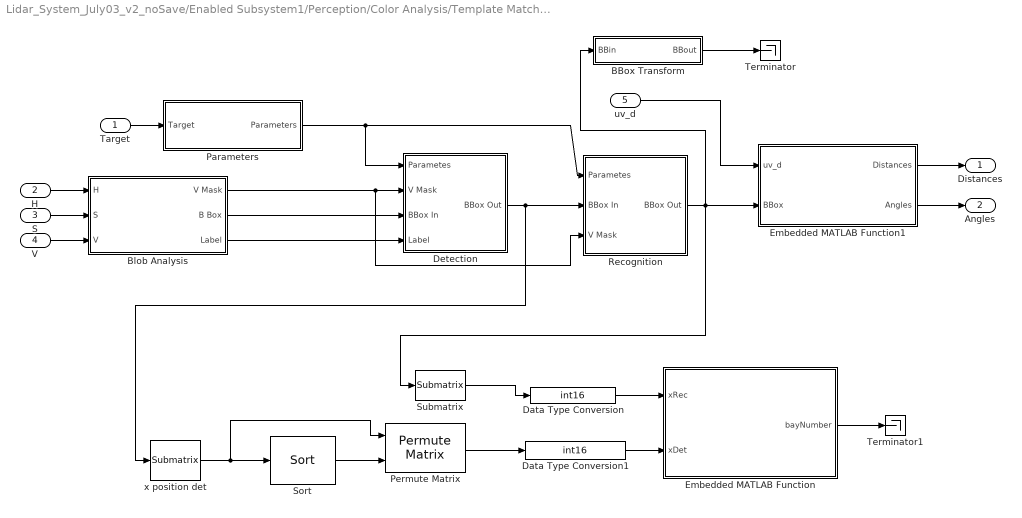
== system Lidar_System_July03_v2_noSave/Enabled Subsystem1/Perception/Color Analysis/Template Matching (Docking)/Black/Circle/Docking1 ==
  Target : Inport
  H : Inport  Port=2
  S : Inport  Port=3
  V : Inport  Port=4
  uv_d : Inport  Port=5
  BBox Transform : Stateflow chart
  Blob Analysis : Subsystem
  Data Type Conversion : DataTypeConversion  OutDataTypeMode=int16  OutDataType=fixdt(1, 16)  OutScaling=2^0  OutDataTypeStr=int16
  Data Type Conversion1 : DataTypeConversion  OutDataTypeMode=int16  OutDataType=fixdt(1, 16)  OutScaling=2^0  OutDataTypeStr=int16
  Detection : Subsystem
  Embedded MATLAB Function : Stateflow chart
  Embedded MATLAB Function1 : Stateflow chart
  Parameters : Subsystem
  Permute Matrix : dspmtrx3/Permute Matrix  mode=Rows  ZeroOneIdxMode=One-based  errmode=Clip index  checkDims=off
  Recognition : Subsystem
  Sort : dspstat3/Sort  DialogController=dspDDGCreate  DialogControllerArgs=DataTag6  otype=Index  dir=Ascending  sortAlg=Quick sort  roundingMode=Floor  overflowMode=off
  Submatrix : dspmtrx3/Submatrix  RowSpan=Range of rows  RowStartMode=First  RowStartIndex=1  RowEndMode=Last  RowEndIndex=1  ColSpan=One column  ColStartMode=First  ColStartIndex=1  ColEndMode=Last  ColEndIndex=1
  Terminator : Terminator
  Terminator1 : Terminator
  x position det : dspmtrx3/Submatrix  RowSpan=Range of rows  RowStartMode=First  RowStartIndex=1  RowEndMode=Last  RowEndIndex=1  ColSpan=One column  ColStartMode=First  ColStartIndex=1  ColEndMode=Last  ColEndIndex=1
  Distances : Outport
  Angles : Outport  Port=2
  wires:
  Embedded MATLAB Function1/2(Angles) -> Angles/1
  BBox Transform/1(BBout) -> Terminator/1
  Target/1 -> Parameters/1(Target)
  V/1 -> Blob Analysis/3(V)
  S/1 -> Blob Analysis/2(S)
  H/1 -> Blob Analysis/1(H)
  Embedded MATLAB Function1/1(Distances) -> Distances/1
  uv_d/1 -> Embedded MATLAB Function1/1(uv_d)
  Embedded MATLAB Function/1(bayNumber) -> Terminator1/1
  Recognition/1(BBox Out) -> BBox Transform/1(BBin), Embedded MATLAB Function1/2(BBox), Submatrix/1
  Data Type Conversion1/1 -> Embedded MATLAB Function/2(xDet)
  Data Type Conversion/1 -> Embedded MATLAB Function/1(xRec)
  Permute Matrix/1 -> Data Type Conversion1/1
  Submatrix/1 -> Data Type Conversion/1
  Sort/1 -> Permute Matrix/2
  x position det/1 -> Permute Matrix/1, Sort/1
  Detection/1(BBox Out) -> x position det/1, Recognition/2(BBox In)
  Blob Analysis/3(Label) -> Detection/4(Label)
  Blob Analysis/2(B Box) -> Detection/3(BBox In)
  Blob Analysis/1(V Mask) -> Recognition/3(V Mask), Detection/2(V Mask)
  Parameters/1(Parameters) -> Recognition/1(Parametes), Detection/1(Parametes)

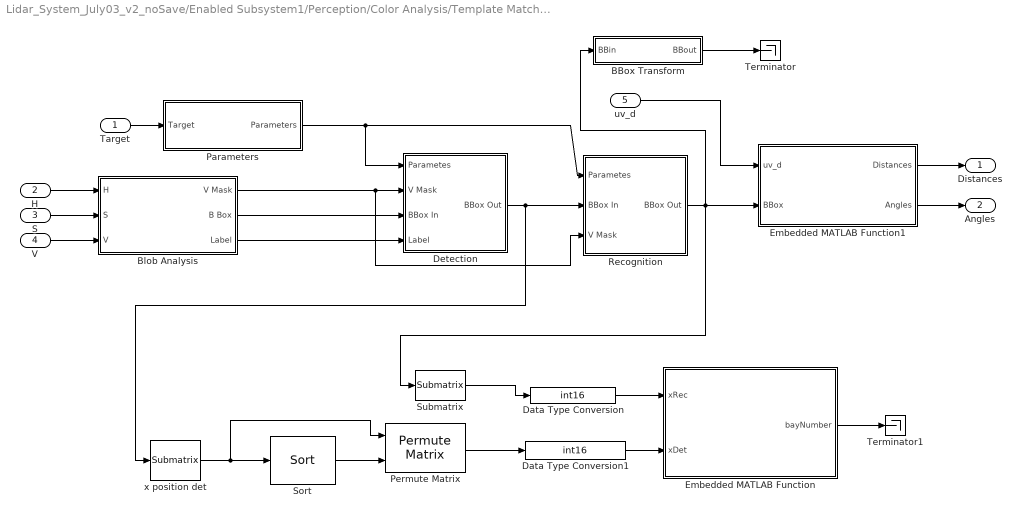
== system Lidar_System_July03_v2_noSave/Enabled Subsystem1/Perception/Color Analysis/Template Matching (Docking)/Black/Cruciform/Docking1 ==
  Target : Inport
  H : Inport  Port=2
  S : Inport  Port=3
  V : Inport  Port=4
  uv_d : Inport  Port=5
  BBox Transform : Stateflow chart
  Blob Analysis : Subsystem
  Data Type Conversion : DataTypeConversion  OutDataTypeMode=int16  OutDataType=fixdt(1, 16)  OutScaling=2^0  OutDataTypeStr=int16
  Data Type Conversion1 : DataTypeConversion  OutDataTypeMode=int16  OutDataType=fixdt(1, 16)  OutScaling=2^0  OutDataTypeStr=int16
  Detection : Subsystem
  Embedded MATLAB Function : Stateflow chart
  Embedded MATLAB Function1 : Stateflow chart
  Parameters : Subsystem
  Permute Matrix : dspmtrx3/Permute Matrix  mode=Rows  ZeroOneIdxMode=One-based  errmode=Clip index  checkDims=off
  Recognition : Subsystem
  Sort : dspstat3/Sort  DialogController=dspDDGCreate  DialogControllerArgs=DataTag10  otype=Index  dir=Ascending  sortAlg=Quick sort  roundingMode=Floor  overflowMode=off
  Submatrix : dspmtrx3/Submatrix  RowSpan=Range of rows  RowStartMode=First  RowStartIndex=1  RowEndMode=Last  RowEndIndex=1  ColSpan=One column  ColStartMode=First  ColStartIndex=1  ColEndMode=Last  ColEndIndex=1
  Terminator : Terminator
  Terminator1 : Terminator
  x position det : dspmtrx3/Submatrix  RowSpan=Range of rows  RowStartMode=First  RowStartIndex=1  RowEndMode=Last  RowEndIndex=1  ColSpan=One column  ColStartMode=First  ColStartIndex=1  ColEndMode=Last  ColEndIndex=1
  Distances : Outport
  Angles : Outport  Port=2
  wires:
  Embedded MATLAB Function1/2(Angles) -> Angles/1
  BBox Transform/1(BBout) -> Terminator/1
  Target/1 -> Parameters/1(Target)
  V/1 -> Blob Analysis/3(V)
  S/1 -> Blob Analysis/2(S)
  H/1 -> Blob Analysis/1(H)
  Embedded MATLAB Function1/1(Distances) -> Distances/1
  uv_d/1 -> Embedded MATLAB Function1/1(uv_d)
  Embedded MATLAB Function/1(bayNumber) -> Terminator1/1
  Recognition/1(BBox Out) -> BBox Transform/1(BBin), Embedded MATLAB Function1/2(BBox), Submatrix/1
  Data Type Conversion1/1 -> Embedded MATLAB Function/2(xDet)
  Data Type Conversion/1 -> Embedded MATLAB Function/1(xRec)
  Permute Matrix/1 -> Data Type Conversion1/1
  Submatrix/1 -> Data Type Conversion/1
  Sort/1 -> Permute Matrix/2
  x position det/1 -> Permute Matrix/1, Sort/1
  Detection/1(BBox Out) -> x position det/1, Recognition/2(BBox In)
  Blob Analysis/3(Label) -> Detection/4(Label)
  Blob Analysis/2(B Box) -> Detection/3(BBox In)
  Blob Analysis/1(V Mask) -> Recognition/3(V Mask), Detection/2(V Mask)
  Parameters/1(Parameters) -> Recognition/1(Parametes), Detection/1(Parametes)

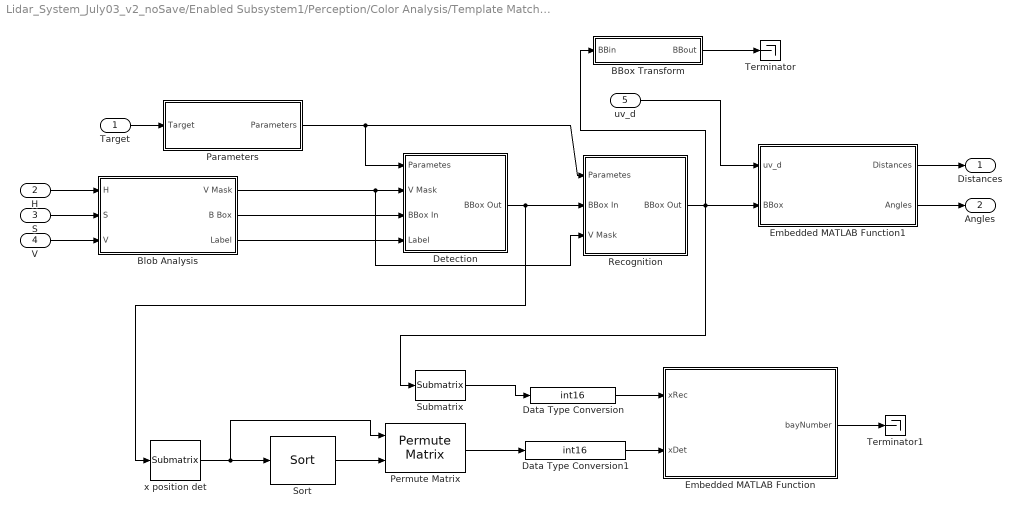
== system Lidar_System_July03_v2_noSave/Enabled Subsystem1/Perception/Color Analysis/Template Matching (Docking)/Black/Triangle/Docking1 ==
  Target : Inport
  H : Inport  Port=2
  S : Inport  Port=3
  V : Inport  Port=4
  uv_d : Inport  Port=5
  BBox Transform : Stateflow chart
  Blob Analysis : Subsystem
  Data Type Conversion : DataTypeConversion  OutDataTypeMode=int16  OutDataType=fixdt(1, 16)  OutScaling=2^0  OutDataTypeStr=int16
  Data Type Conversion1 : DataTypeConversion  OutDataTypeMode=int16  OutDataType=fixdt(1, 16)  OutScaling=2^0  OutDataTypeStr=int16
  Detection : Subsystem
  Embedded MATLAB Function : Stateflow chart
  Embedded MATLAB Function1 : Stateflow chart
  Parameters : Subsystem
  Permute Matrix : dspmtrx3/Permute Matrix  mode=Rows  ZeroOneIdxMode=One-based  errmode=Clip index  checkDims=off
  Recognition : Subsystem
  Sort : dspstat3/Sort  DialogController=dspDDGCreate  DialogControllerArgs=DataTag14  otype=Index  dir=Ascending  sortAlg=Quick sort  roundingMode=Floor  overflowMode=off
  Submatrix : dspmtrx3/Submatrix  RowSpan=Range of rows  RowStartMode=First  RowStartIndex=1  RowEndMode=Last  RowEndIndex=1  ColSpan=One column  ColStartMode=First  ColStartIndex=1  ColEndMode=Last  ColEndIndex=1
  Terminator : Terminator
  Terminator1 : Terminator
  x position det : dspmtrx3/Submatrix  RowSpan=Range of rows  RowStartMode=First  RowStartIndex=1  RowEndMode=Last  RowEndIndex=1  ColSpan=One column  ColStartMode=First  ColStartIndex=1  ColEndMode=Last  ColEndIndex=1
  Distances : Outport
  Angles : Outport  Port=2
  wires:
  Embedded MATLAB Function1/2(Angles) -> Angles/1
  BBox Transform/1(BBout) -> Terminator/1
  Target/1 -> Parameters/1(Target)
  V/1 -> Blob Analysis/3(V)
  S/1 -> Blob Analysis/2(S)
  H/1 -> Blob Analysis/1(H)
  Embedded MATLAB Function1/1(Distances) -> Distances/1
  uv_d/1 -> Embedded MATLAB Function1/1(uv_d)
  Embedded MATLAB Function/1(bayNumber) -> Terminator1/1
  Recognition/1(BBox Out) -> BBox Transform/1(BBin), Embedded MATLAB Function1/2(BBox), Submatrix/1
  Data Type Conversion1/1 -> Embedded MATLAB Function/2(xDet)
  Data Type Conversion/1 -> Embedded MATLAB Function/1(xRec)
  Permute Matrix/1 -> Data Type Conversion1/1
  Submatrix/1 -> Data Type Conversion/1
  Sort/1 -> Permute Matrix/2
  x position det/1 -> Permute Matrix/1, Sort/1
  Detection/1(BBox Out) -> x position det/1, Recognition/2(BBox In)
  Blob Analysis/3(Label) -> Detection/4(Label)
  Blob Analysis/2(B Box) -> Detection/3(BBox In)
  Blob Analysis/1(V Mask) -> Recognition/3(V Mask), Detection/2(V Mask)
  Parameters/1(Parameters) -> Recognition/1(Parametes), Detection/1(Parametes)
